simulink model "neurosin"  (Simulink 8.3)
settings: Solver=ode3  StartTime=0.0  StopTime=1500  FixedStep=0.3  MinStep=0.3  RelTol=1e-3
libraries: simulink x3
settings Model: Creator=Administrator  LastModifiedBy=jackyjing
settings OptimizationCC: ExpressionDepthLimit=2147483647
settings DebuggingCC: FcnCallInpInsideContextMsg=UseLocalSettings

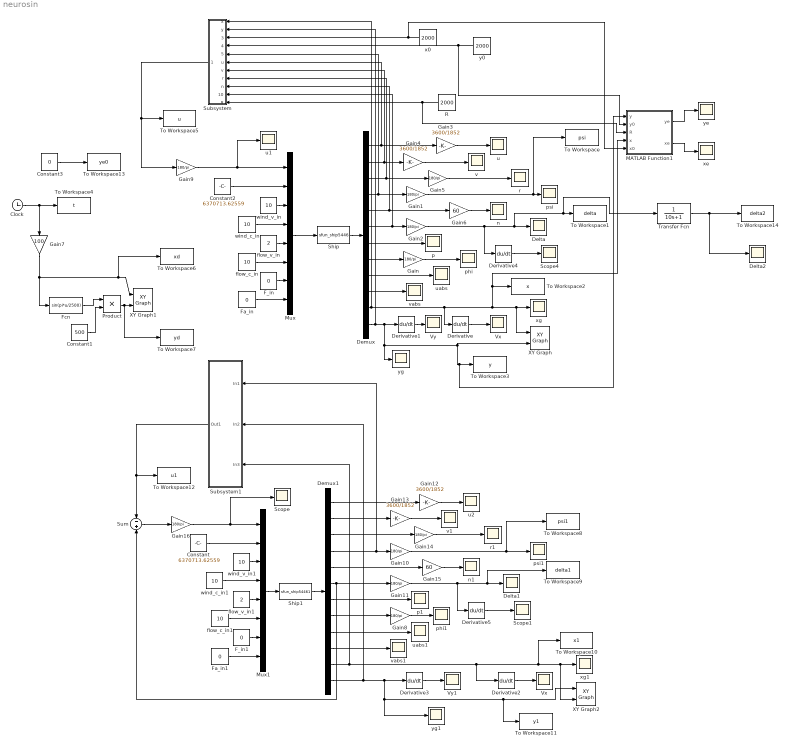
== system neurosin ==
  Clock : Clock
  Constant : Constant  Value=6370713.62559
  Constant1 : Constant  Value=500
  Constant2 : Constant  Value=6370713.62559
  Constant3 : Constant  Value=0
  Delta : Scope
      settings: TickLabels=on  TimeRange=1500  YMin=-27.5  YMax=20  SaveName=ScopeData5
  Delta1 : Scope
      settings: TickLabels=on  TimeRange=1500  YMin=-35  YMax=35  SaveName=ScopeData29
  Delta2 : Scope
      settings: TickLabels=on  TimeRange=1500  YMin=-30  YMax=20  SaveName=ScopeData45
  Demux : Demux  Outputs=12
  Demux1 : Demux  Outputs=12
  Derivative{,1..5} (6 alike) : Derivative
  F_in : Constant  Value=0
  F_in1 : Constant  Value=0
  Fa_in : Constant  Value=0
  Fa_in1 : Constant  Value=0
  Fcn : Fcn  Expr=sin(pi*u/2500)
  Gain{,1..2,5,8..11,14,16} (10 alike) : Gain  Gain=180/pi
  Gain{3..4,12..13} (4 alike) : Gain  Gain=3600/1852
  Gain15 : Gain  Gain=60
  Gain6 : Gain  Gain=60
  Gain7 : Gain  Gain=100
  MATLAB Function1 : MATLAB Function  TreatAsAtomicUnit=on
  Mux : Mux  Inputs=8
  Mux1 : Mux  Inputs=8
  Product : Product
  R : Constant  Value=2000
  Scope : Scope
      settings: TimeRange=1000  YMin=-0.6  YMax=0.8  SaveName=ScopeData30
  Scope1 : Scope
      settings: YMin=-0.005  YMax=0.002  SaveName=ScopeData31
  Scope4 : Scope
      settings: YMin=-0.005  YMax=0.002  SaveName=ScopeData18
  Ship : S-Function  FunctionName=sfun_ship5446  EnableBusSupport=off
  Ship1 : S-Function  FunctionName=sfun_ship54461  EnableBusSupport=off
  Subsystem : Subsystem
  Subsystem1 : Subsystem
  Sum : Sum  Inputs=-|+
  To Workspace : ToWorkspace  VariableName=psi  SampleTime=-1
  To Workspace1 : ToWorkspace  VariableName=delta  SampleTime=-1
  To Workspace10 : ToWorkspace  VariableName=x1  SampleTime=-1
  To Workspace11 : ToWorkspace  VariableName=y1  SampleTime=-1
  To Workspace12 : ToWorkspace  VariableName=u1  SampleTime=-1
  To Workspace13 : ToWorkspace  VariableName=ye0  SampleTime=-1
  To Workspace14 : ToWorkspace  VariableName=delta2  SampleTime=-1
  To Workspace2 : ToWorkspace  VariableName=x  SampleTime=-1
  To Workspace3 : ToWorkspace  VariableName=y  SampleTime=-1
  To Workspace4 : ToWorkspace  VariableName=t  SampleTime=-1
  To Workspace5 : ToWorkspace  VariableName=u  SampleTime=-1
  To Workspace6 : ToWorkspace  VariableName=xd  SampleTime=-1
  To Workspace7 : ToWorkspace  VariableName=yd  SampleTime=-1
  To Workspace8 : ToWorkspace  VariableName=psi1  SampleTime=-1
  To Workspace9 : ToWorkspace  VariableName=delta1  SampleTime=-1
  Transfer Fcn : TransferFcn  Denominator=[10 1]
  Vx : Scope
      settings: TickLabels=on  SaveName=ScopeData8
  "Vx " : Scope
      settings: TickLabels=on  SaveName=ScopeData32
  Vy : Scope
      settings: TickLabels=on  SaveName=ScopeData9
  Vy1 : Scope
      settings: TickLabels=on  SaveName=ScopeData33
  XY Graph : simulink/Sinks/XY Graph  xmin=-1000  xmax=20000  ymin=-2000  ymax=2000  st=-1
  XY Graph1 : simulink/Sinks/XY Graph  xmin=-1000  xmax=20000  ymin=-2000  ymax=2000  st=-1
  XY Graph2 : simulink/Sinks/XY Graph  xmin=-1000  xmax=20000  ymin=-2000  ymax=2000  st=-1
  flow_c_in : Constant  Value=10
  flow_c_in1 : Constant  Value=10
  flow_v_in : Constant  Value=2
  flow_v_in1 : Constant  Value=2
  n : Scope
      settings: TickLabels=on  YMin=38.5  YMax=46.5  SaveName=ScopeData4
  n1 : Scope
      settings: TickLabels=on  YMin=38.5  YMax=46.5  SaveName=ScopeData34
  p : Scope
      settings: TickLabels=on  SaveName=ScopeData10
  p1 : Scope
      settings: TickLabels=on  SaveName=ScopeData35
  phi : Scope
      settings: YMin=-0.00175  YMax=0.0015  SaveName=ScopeData11
  phi1 : Scope
      settings: YMin=-0.00175  YMax=0.0015  SaveName=ScopeData36
  psi : Scope
      settings: TickLabels=on  TimeRange=44.44444444444434  YMin=52  YMax=60.5  SaveName=ScopeData3
  psi1 : Scope
      settings: TickLabels=on  TimeRange=500  YMin=9.9825  YMax=10.01  SaveName=ScopeData37
  r : Scope
      settings: TickLabels=on  SaveName=ScopeData2
  r1 : Scope
      settings: TickLabels=on  SaveName=ScopeData38
  u : Scope
      settings: TickLabels=on  YMin=28.45  YMax=29.45
  u1 : Scope
      settings: TickLabels=on  TimeRange=1500  YMin=-35000  YMax=35000  SaveName=ScopeData15
  u2 : Scope
      settings: TickLabels=on  YMin=15.075  YMax=15.625  SaveName=ScopeData39
  uabs : Scope
      settings: TickLabels=on  YMin=10.75  YMax=15  SaveName=ScopeData6
  uabs1 : Scope
      settings: TickLabels=on  YMin=10.75  YMax=15  SaveName=ScopeData40
  v : Scope
      settings: TickLabels=on
  v1 : Scope
      settings: TickLabels=on  YMin=-0.3  YMax=0.15  SaveName=ScopeData41
  vabs : Scope
      settings: TickLabels=on  YMin=-1.75  YMax=0  SaveName=ScopeData7
  vabs1 : Scope
      settings: TickLabels=on  YMin=-1.75  YMax=0  SaveName=ScopeData42
  wind_c_in : Constant  Value=10
  wind_c_in1 : Constant  Value=10
  wind_v_in : Constant  Value=10
  wind_v_in1 : Constant  Value=10
  x0 : Constant  Value=2000
  xe : Scope
      settings: TickLabels=on  YMin=-475  YMax=50  SaveName=ScopeData16
  xg : Scope
      settings: TickLabels=on  YMin=250  YMax=475  SaveName=ScopeData12
  xg1 : Scope
      settings: TickLabels=on  YMin=-300  YMax=900  SaveName=ScopeData43
  y0 : Constant  Value=2000
  ye : Scope
      settings: TickLabels=on  YMin=-550  YMax=250  SaveName=ScopeData17
  yg : Scope
      settings: TickLabels=on  YMin=250  YMax=475  SaveName=ScopeData13
  yg1 : Scope
      settings: TickLabels=on  YMin=250  YMax=475  SaveName=ScopeData44
  wires:
  Ship/1 -> Demux/1
  Demux/1 -> Subsystem/6(u), Gain3/1
  Demux/2 -> Subsystem/7(v), Gain4/1
  Demux/3 -> Subsystem/8(r), Gain5/1
  Demux/5 -> Subsystem/9(n), Gain6/1
  Demux/7 -> p/1
  Demux/8 -> Gain/1
  Demux/4 -> Gain1/1, Subsystem/5(psi)
  Gain/1 -> phi/1
  Gain2/1 -> Derivative4/1, Delta/1, Transfer Fcn/1, To Workspace1/1
  Gain3/1 -> u/1
  Gain4/1 -> v/1
  Gain5/1 -> r/1
  Gain6/1 -> n/1
  Demux/9 -> uabs/1
  Demux/10 -> vabs/1
  Demux/12 -> Subsystem/2(y), Derivative1/1, yg/1, MATLAB Function1/1(y), To Workspace3/1, XY Graph/2
  Demux/11 -> Subsystem/1(x), Derivative/1, XY Graph/1, xg/1, MATLAB Function1/4(x), To Workspace2/1
  Derivative/1 -> Vx/1
  Derivative1/1 -> Vy/1
  wind_v_in/1 -> Mux/3
  wind_c_in/1 -> Mux/4
  flow_v_in/1 -> Mux/5
  F_in/1 -> Mux/7
  Fa_in/1 -> Mux/8
  flow_c_in/1 -> Mux/6
  Mux/1 -> Ship/1
  Constant2/1 -> Mux/2
  Derivative4/1 -> Scope4/1
  Clock/1 -> Gain7/1, To Workspace4/1
  y0/1 -> MATLAB Function1/2(y0), Subsystem/4(y0)
  R/1 -> MATLAB Function1/3(R), Subsystem/11(R)
  Demux/6 -> Subsystem/10(Delta), Gain2/1
  Subsystem/1("psi ") -> Gain9/1, To Workspace5/1
  MATLAB Function1/2(xe) -> xe/1
  MATLAB Function1/1(ye) -> ye/1
  x0/1 -> MATLAB Function1/5(x0), Subsystem/3(x0)
  Gain1/1 -> psi/1, To Workspace/1
  Gain9/1 -> u1/1, Mux/1
  Product/1 -> To Workspace7/1, XY Graph1/2
  Fcn/1 -> Product/1
  Constant1/1 -> Product/2
  Gain7/1 -> To Workspace6/1, XY Graph1/1, Fcn/1
  Ship1/1 -> Demux1/1
  Demux1/1 -> Gain12/1
  Demux1/2 -> Gain13/1
  Demux1/3 -> Gain14/1
  Demux1/5 -> Gain15/1
  Demux1/6 -> Sum/2, Gain11/1
  Demux1/7 -> p1/1
  Demux1/8 -> Gain8/1
  Gain10/1 -> psi1/1, To Workspace8/1
  Gain8/1 -> phi1/1
  Gain12/1 -> u2/1
  Gain13/1 -> v1/1
  Gain14/1 -> r1/1
  Gain15/1 -> n1/1
  Demux1/9 -> uabs1/1
  Demux1/10 -> vabs1/1
  Demux1/12 -> Derivative3/1, yg1/1, XY Graph2/1, To Workspace11/1, Subsystem1/2(In2)
  Demux1/11 -> Subsystem1/3(In3), Derivative2/1, xg1/1, XY Graph2/2, To Workspace10/1
  Derivative2/1 -> "Vx "/1
  Derivative3/1 -> Vy1/1
  wind_v_in1/1 -> Mux1/3
  wind_c_in1/1 -> Mux1/4
  flow_v_in1/1 -> Mux1/5
  F_in1/1 -> Mux1/7
  Fa_in1/1 -> Mux1/8
  flow_c_in1/1 -> Mux1/6
  Mux1/1 -> Ship1/1
  Constant/1 -> Mux1/2
  Sum/1 -> Gain16/1
  Derivative5/1 -> Scope1/1
  Subsystem1/1(Out1) -> Sum/1, To Workspace12/1
  Demux1/4 -> Gain10/1, Subsystem1/1(In1)
  Gain11/1 -> Derivative5/1, Delta1/1, To Workspace9/1
  Gain16/1 -> Mux1/1, Scope/1
  Constant3/1 -> To Workspace13/1
  Transfer Fcn/1 -> Delta2/1, To Workspace14/1

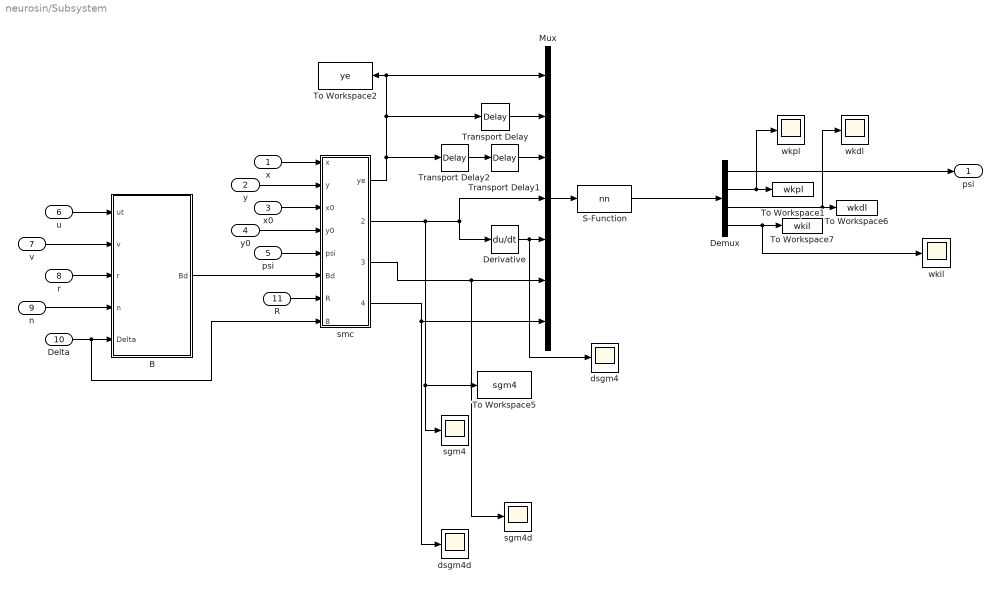
== system neurosin/Subsystem ==
  x : Inport
  y : Inport  Port=2
  x0 : Inport  Port=3
  y0 : Inport  Port=4
  psi : Inport  Port=5
  u : Inport  Port=6
  v : Inport  Port=7
  r : Inport  Port=8
  n : Inport  Port=9
  Delta : Inport  Port=10
  R : Inport  Port=11
  B : MATLAB Function  TreatAsAtomicUnit=on
  Demux : Demux
  Derivative : Derivative
  Mux : Mux  Inputs=7
  S-Function : S-Function  FunctionName=nn  EnableBusSupport=off
  To Workspace1 : ToWorkspace  VariableName=wkpl  SampleTime=-1
  To Workspace2 : ToWorkspace  VariableName=ye  SampleTime=-1
  To Workspace5 : ToWorkspace  VariableName=sgm4  SampleTime=-1
  To Workspace6 : ToWorkspace  VariableName=wkdl  SampleTime=-1
  To Workspace7 : ToWorkspace  VariableName=wkil  SampleTime=-1
  Transport Delay : TransportDelay  DelayTime=2
  Transport Delay1 : TransportDelay
  Transport Delay2 : TransportDelay
  dsgm4 : Scope
      settings: TickLabels=on  TimeRange=1500  YMin=-4.20046e+11  YMax=-3.80042e+11  SaveName=ScopeData25
  dsgm4d : Scope
      settings: TickLabels=on  TimeRange=1500  YMin=0.00019  YMax=0.00028  SaveName=ScopeData23
  sgm4 : Scope
      settings: TickLabels=on  TimeRange=1500  YMin=-0.002  YMax=0.002  SaveName=ScopeData24
  sgm4d : Scope
      settings: TickLabels=on  TimeRange=1500  YMin=0.00975  YMax=0.014  SaveName=ScopeData21
  "smc " : Subsystem
  wkdl : Scope
      settings: TickLabels=on  TimeRange=1500  YMin=-2.5e+08  YMax=2.5e+09  SaveName=ScopeData19
  wkil : Scope
      settings: TickLabels=on  TimeRange=1500  YMin=-3e+08  YMax=2.5e+07  SaveName=ScopeData20
  wkpl : Scope
      settings: TickLabels=on  TimeRange=1500  YMin=-3.75e+10  YMax=2.5e+09  SaveName=ScopeData22
  "psi " : Outport
  wires:
  x/1 -> "smc "/1(x)
  y/1 -> "smc "/2(y)
  x0/1 -> "smc "/3(x0)
  y0/1 -> "smc "/4(y0)
  psi/1 -> "smc "/5("psi ")
  u/1 -> B/1(ut)
  v/1 -> B/2(v)
  r/1 -> B/3(r)
  n/1 -> B/4(n)
  Mux/1 -> S-Function/1
  Transport Delay/1 -> Mux/2
  Transport Delay1/1 -> Mux/3
  Derivative/1 -> dsgm4/1, Mux/5
  B/1(Bd) -> "smc "/6(Bd)
  Transport Delay2/1 -> Transport Delay1/1
  R/1 -> "smc "/7(R)
  Delta/1 -> "smc "/8(delta), B/5(Delta)
  S-Function/1 -> Demux/1
  Demux/2 -> To Workspace1/1, wkpl/1
  Demux/3 -> To Workspace6/1, wkdl/1
  Demux/4 -> wkil/1, To Workspace7/1
  Demux/1 -> "psi "/1
  "smc "/1(ye) -> Transport Delay2/1, Transport Delay/1, Mux/1, To Workspace2/1
  "smc "/2(sgm4) -> Mux/4, Derivative/1, To Workspace5/1, sgm4/1
  "smc "/3(sgm4d) -> sgm4d/1, Mux/6
  "smc "/4(dsgm4d) -> Mux/7, dsgm4d/1

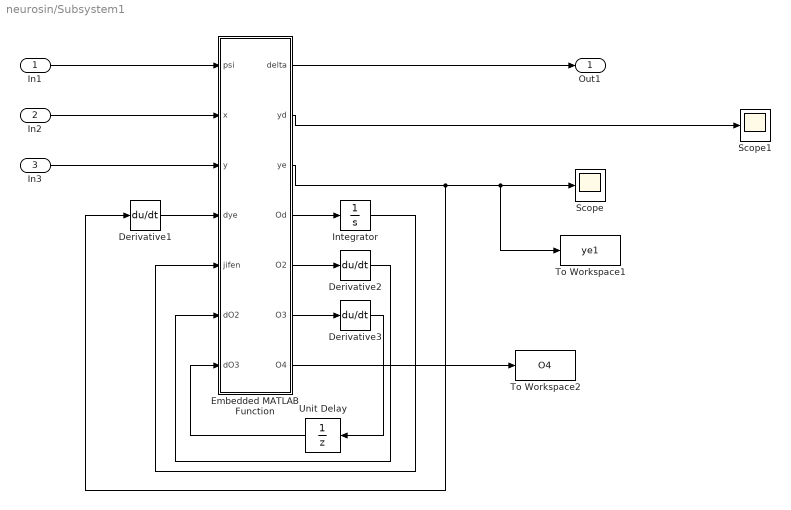
== system neurosin/Subsystem1 ==
  In1 : Inport
  In2 : Inport  Port=2
  In3 : Inport  Port=3
  Derivative1 : Derivative
  Derivative2 : Derivative
  Derivative3 : Derivative
  Embedded MATLAB Function : MATLAB Function  TreatAsAtomicUnit=on
  Integrator : Integrator
  Scope : Scope
      settings: YMin=-50  YMax=750  SaveName=ScopeData16
  Scope1 : Scope
      settings: YMin=-700  YMax=700  SaveName=ScopeData17
  To Workspace1 : ToWorkspace  VariableName=ye1  SampleTime=-1
  To Workspace2 : ToWorkspace  VariableName=O4  SampleTime=-1
  Unit Delay : UnitDelay  SampleTime=-1
  Out1 : Outport
  wires:
  Embedded MATLAB Function/6(O3) -> Derivative3/1
  Derivative3/1 -> Unit Delay/1
  Embedded MATLAB Function/5(O2) -> Derivative2/1
  Derivative2/1 -> Embedded MATLAB Function/6(dO2)
  Integrator/1 -> Embedded MATLAB Function/5(jifen)
  Embedded MATLAB Function/1(delta) -> Out1/1
  Embedded MATLAB Function/4(Od) -> Integrator/1
  In1/1 -> Embedded MATLAB Function/1(psi)
  In2/1 -> Embedded MATLAB Function/2(x)
  In3/1 -> Embedded MATLAB Function/3(y)
  Embedded MATLAB Function/3(ye) -> Derivative1/1, To Workspace1/1, Scope/1
  Derivative1/1 -> Embedded MATLAB Function/4(dye)
  Unit Delay/1 -> Embedded MATLAB Function/7(dO3)
  Embedded MATLAB Function/2(yd) -> Scope1/1
  Embedded MATLAB Function/7(O4) -> To Workspace2/1

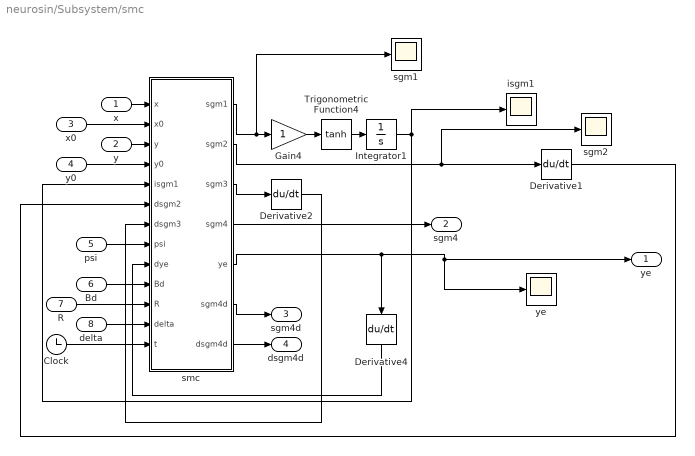
== system neurosin/Subsystem/smc  ==
  x : Inport
  y : Inport  Port=2
  x0 : Inport  Port=3
  y0 : Inport  Port=4
  "psi " : Inport  Port=5
  Bd : Inport  Port=6
  R : Inport  Port=7
  delta : Inport  Port=8
  Clock : Clock
  Derivative1 : Derivative
  Derivative2 : Derivative
  Derivative4 : Derivative
  Gain4 : Gain
  Integrator1 : Integrator
  Trigonometric Function4 : Trigonometry  Operator=tanh
  isgm1 : Scope
      settings: TickLabels=on  TimeRange=1500  YMin=-150  YMax=650  SaveName=ScopeData28
  sgm1 : Scope
      settings: TickLabels=on  TimeRange=1500  YMin=-15  YMax=15  SaveName=ScopeData26
  sgm2 : Scope
      settings: TickLabels=on  TimeRange=1500  YMax=7  SaveName=ScopeData27
  "smc " : MATLAB Function  TreatAsAtomicUnit=on
  "ye " : Scope
      settings: TimeRange=1500  YMin=-17.5  YMax=22.5  SaveName=ScopeData14
  ye : Outport
  sgm4 : Outport  Port=2
  sgm4d : Outport  Port=3
  dsgm4d : Outport  Port=4
  wires:
  "smc "/1(sgm1) -> sgm1/1, Gain4/1
  Derivative2/1 -> "smc "/7(dsgm3)
  "smc "/3(sgm3) -> Derivative2/1
  Trigonometric Function4/1 -> Integrator1/1
  Derivative1/1 -> "smc "/6(dsgm2)
  Integrator1/1 -> isgm1/1, "smc "/5(isgm1)
  x/1 -> "smc "/1(x)
  y/1 -> "smc "/3(y)
  x0/1 -> "smc "/2(x0)
  y0/1 -> "smc "/4(y0)
  "smc "/4(sgm4) -> sgm4/1
  "smc "/5(ye) -> "ye "/1, ye/1, Derivative4/1
  Bd/1 -> "smc "/10(Bd)
  Derivative4/1 -> "smc "/9(dye)
  "smc "/6(sgm4d) -> sgm4d/1
  "smc "/7(dsgm4d) -> dsgm4d/1
  R/1 -> "smc "/11(R)
  delta/1 -> "smc "/12(delta)
  Gain4/1 -> Trigonometric Function4/1
  "psi "/1 -> "smc "/8(psi)
  "smc "/2(sgm2) -> Derivative1/1, sgm2/1
  Clock/1 -> "smc "/13(t)

== matlab function Subsystem/smc /smc  ==
  data: x input double; x0 input double; y input double; y0 input double; isgm1 input double; dsgm2 input double; dsgm3 input double; sgm1 output double; sgm2 output double; sgm3 output double; psi input double; dye input double; sgm4 output double; ye output double; Bd input double; sgm4d output double; dsgm4d output double; R input double; delta input double; t input double
function [sgm1,sgm2,sgm3,sgm4,ye,sgm4d,dsgm4d]= fcn(x,x0,y,y0,isgm1,dsgm2,dsgm3,psi,dye,Bd,R,delta,t)
%#codegen
k0=0.01;k1=3;k2=0.02;k3=0.005;k4=0.01;

 ye=y-500*sin(pi*x/2500);

sgm1=k1*tanh(k0*ye)+dye;
sgm2=psi+k2*isgm1;
sgm3=k3*tanh(sgm2)+dsgm2;
sgm4=k4*tanh(sgm3)+dsgm3;

sgm4d=Bd; 
dsgm4d=(k4*(sech(sgm3)^2)+k3*(sech(sgm2)^2))*Bd;

== matlab function Subsystem/B ==
  data: ut input double; Bd output double; v input double; r input double; n input double; Delta input double
function Bd  = fcn(ut,v,r,n,Delta)
% function ud = fcn(ut,v,r,n,Delta,phi,dr,sgm4)
V=sqrt(ut*ut+v*v);%u=x(1) v=x(2)

da=10.5;%9.34+0.25;%尾吃水13.8;%12.5;%
df=7.5;%4.97+0.25;%首吃水14.3;%13.8;%
Dh=9.0;%舵高s   ;%11.411.4;;%+7.00+0.25
pa=1.205;%%%**空气密度
Lpp=267.0;%船长
B=39.8;%船宽
Db=6.466;%舵宽
P=9.657;%da螺距
luow=1026;%小luow是密度 水密度
Dp=9.2;%螺旋桨直径
Ds=23.6;%型深
d=(da+df)/2;%吃水
m=(165.89*d*d + 4383.9*d)*1000;%排水量
Cb=m/(Lpp*B*d*1.025*1000);
AR=(d-7.41)/(12.5-7.41)*(81.44-43.14)+43.14;%舵叶面积
d_B=d/B;L_B=Lpp/B;
mx=m/100*(0.398+11.97*Cb*(1+3.73*d_B)-2.89*Cb*L_B*(1+1.13*d_B)+0.175*Cb*L_B*L_B*(1+0.541*d_B)-1.107*L_B*d_B);
my=m*(0.882-0.54*Cb*(1-1.6*d_B)-0.156*L_B*(1-0.673*Cb)+0.826*d_B*L_B*(1-0.678*d_B)-0.638*Cb*d_B*L_B*(1-0.669*d_B));
wp0=0.5*Cb-0.05;
fa=6.13*Dh/Db/(2.25+Dh/Db);
gma=-22.2*(Cb*B/Lpp)*(Cb*B/Lpp)+0.02*(Cb*B/Lpp)+0.68;
gmaR=1.1633-1.98828*Cb+1.3902*Cb*Cb;
tR=0.7382-0.0539*Cb+0.1755*Cb*Cb;
ifaH=0.6784-1.3374*Cb+1.8891*Cb*Cb;
xH=-(0.4+0.1*Cb)*Lpp;
xR=-0.5*Lpp;
xb=1.87;
Jzz=1/100.0*(33-76.85*Cb*(1-0.784*Cb)+3.43*L_B*(1-0.63*Cb))*Lpp*Lpp;
Izz=(1.0+(Cb^4.5))*m*(Lpp*Lpp+power(B,2.4))/24.0;

m33=Izz+Jzz;

beta=atan2((-v),(ut));%u=x(1) v=x(2)
betap=beta+0.5*r*Lpp/V;%r=x(3)
betaR=beta+r*Lpp/V;
wp=wp0*exp(-4.0*betap*betap);
up=(1.0-wp)*ut;%u=x(1)
s=1.0-up/n/P;% n=x(5)
eta=Dp/Dh;

k=0.6;
Gs=eta*k*(2.0-(2.0-k)*s)*s/(1.0-s)/(1.0-s);
s0=1-(1-wp0)*ut/n/P;% n=x(5)u=x(1)
delt0=-s0/57.3;

if(Delta<0)
    K=1.065;
else
    K=0.935;
end
%
uR=up*(1+K*Gs)^0.5;
vRp=uR*delt0;
vR=vRp-gmaR*(v-Lpp*r);%r=x(3)v=x(2)
UR2=uR*uR+vR*vR;
J=ut*(1-wp)/n/Dp;%u=x(1)  n=x(5)
if(J<=0.3)
    L_ifaH=ifaH*J/0.3;% p137, 3-5-119
else
    L_ifaH=ifaH;
end
%
Bd=(-1.0/2.0)*(xR+L_ifaH*xH)*luow*AR*fa*UR2*cos(Delta)/(m33);

== matlab function Subsystem1/Embedded MATLAB Function ==
  data: psi input double; x input double; y input double; dye input double; delta output double; yd output double; ye output double; Od output double; O2 output double; O3 output double; jifen input double; dO2 input double; dO3 input double; O4 output double
function [delta,yd,ye,Od,O2,O3,O4] = fcn(psi,x,y,dye,jifen,dO2,dO3)

K0=0.001;K1=15;K2=1;K3=0.0005;K4=0.02;K5=20000;Te=2.5;

% K0=0.001;K1=15;K2=1;K3=0.0005;K4=0.02;K5=1;Te=2.5;

yd=500*sin(pi*x/2500);
ye=y-yd;


O1=K1*f(K0*ye)+dye;
Od=f(O1);
O2=psi+K2*jifen;
O3=K3*f(O2)+dO2;
O4=K4*f(O3)+dO3;
delta=-Te*K5*O4;

function mean=f(a)
mean=tanh(a);
% function mean=f(a)
% if(a<0.1&&a>-0.1)
%     mean=a;
% else 
%  mean=coth(a)-1/a;
% end

== matlab function MATLAB Function1 ==
  data: y input double; ye output double; y0 input double; R input double; x input double; x0 input double; xe output double
function [ye,xe]= fcn(y,y0,R,x,x0)
%#codegen

thta=atan2((y-y0),(x-x0));
xe = x-x0-R*cos(thta);
ye = y-y0-R*sin(thta);
